simulink model "Convolution_Stream_Ex2"  (R2025a)
settings: Solver=ode4  StopTime=10
undefined symbols (not defined in the file): S, Valid, vsva2197, xcvc1902
libraries: aieUtilities x2, aieDSP x1, vmcUtilities x1
settings Model: Creator=sais  LastModifiedBy=robg

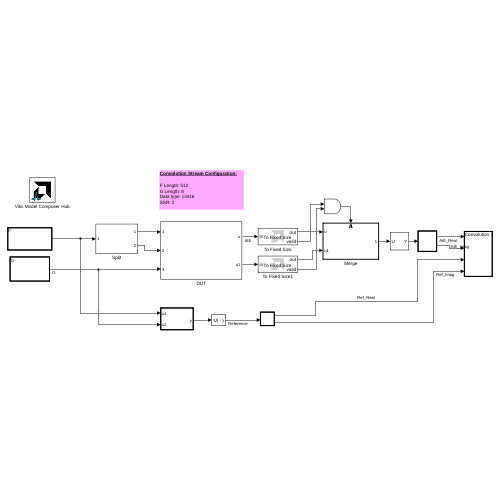
[thumbnail: Simulink's stored preview of the top-level diagram]
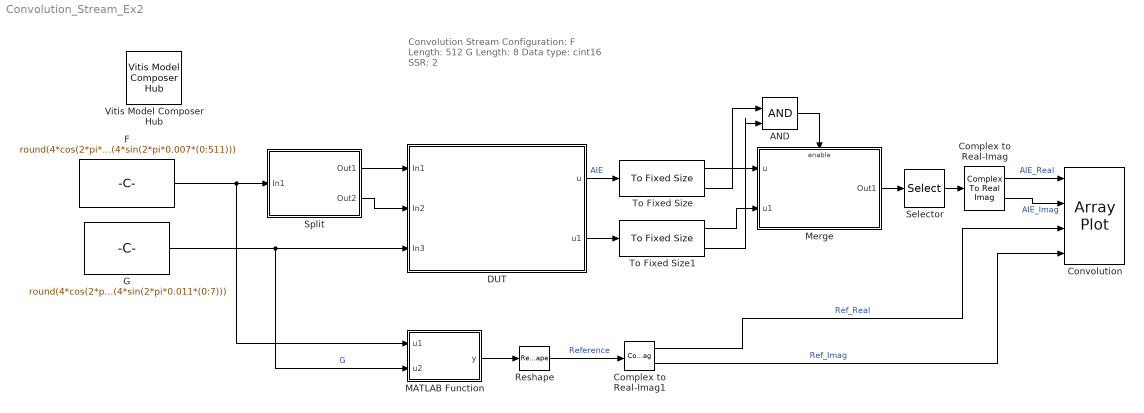
== system Convolution_Stream_Ex2 ==
  note: Convolution Stream Configuration:
      |
      | F Length: 512
      | G Length: 8
      | Data type: cint16
      | SSR: 2
  AND : Logic  IconShape=distinctive  AllPortsSameDT=off  OutDataTypeStr=boolean
  Complex to Real-Imag : ComplexToRealImag
  Complex to Real-Imag1 : ComplexToRealImag
  Convolution : ArrayPlot  NumInputPorts=4  WindowPosition=[379.000000,271.000000,1269.000000,725.000000,]  Visible=on  ScopeFrameLocation=window  YLimits=[-185 185]  ShowLegend=on
  DUT : Subsystem
  F : Constant  Value=round(4*cos(2*pi*0.013*(0:511))) + 1i*round(4*sin(2*pi*0.007*(0:511)))  OutDataTypeStr=int16  SampleTime=1
  G : Constant  Value=round(4*cos(2*pi*0.02*(0:7))) + 1i*round(4*sin(2*pi*0.011*(0:7)))  VectorParams1D=off  OutDataTypeStr=int16  SampleTime=1
  MATLAB Function : MATLAB Function  TreatAsAtomicUnit=on
  Merge : Subsystem
  Reshape : Reshape
  Selector : Selector  InputPortWidth=512  IndexOptions=Index vector (dialog)  Indices=1:1:512-8+1  OutputSizes=1
  Split : Subsystem
  To Fixed Size : aieUtilities/To Fixed Size  Mode=Produce a valid output signal  OutputSize=Inherit: Same as input  CopyMethod=Buffer samples to form output  HasStatusOutput=on
  To Fixed Size1 : aieUtilities/To Fixed Size  Mode=Produce a valid output signal  OutputSize=Inherit: Same as input  CopyMethod=Buffer samples to form output  HasStatusOutput=on
  Vitis Model Composer Hub : vmcUtilities/Vitis Model Composer Hub  Tag=genX  CodeGeneration=off  SubsystemName=DUT  BlockHierPath=Convolution_Stream_Ex2/DUT  CompilationType=HDLCompilation  SubsystemType=DUTNode  ExportTypeV2=IP Catalog  AIEArrayConfig=Use entire AIE array  StartColumn=1  NumberOfColumns=1  TargetDirectory=./code_2iterations  exportDesign=off  analyzeDesign=on  validateDesignOnHw=off  ExportType=AI Engines  IpVendor=xilinx.com  IpLibrary=hls  IpVersion=1.0  IpHWLanguage=Verilog  AieCompilerOptions={}  AieSimulatorOptions={}  CreateTestbench=on  TestbenchStackSize=10  RunRtlSim=off  RunCSim=off  RunAieSim=off  enableSimulationTimeout=on  enableGraphIterations=on  AieSimTimeout=50000  AieGraphIterations=-1  RunAieSimProfiling=off  LaunchVitisAnalyzer=off  PlotOutput=off  RunX86Sim=off  X86SimTimeout=10  GenHwImage=off  GenLibadfXo=off  GenHwValidationCode=off  PlatformType=Not Specified  HwSystemType=Baremetal  HwValidationTarget=hw  ProjDevice=xcvc1902-vsva2197-1LP-e-S  ProjDevicePart=xcvc1902-vsva2197-1LP-e-S  AIEType=AIE  SamplePeriod=-1  ClockFrequency=200  DataPathParallelism=1  xilinxfamily=versalaicore  part=xcvc1902  speed=-1LP-e-S  package=vsva2197  directory=./netlist  testbench=off  incr_netlist=off  synthesis_tool=Vivado  clock_wrapper=Clock Enables  dbl_ovrd=According to Block Masks  dcm_input_clock_period=10  sysclk_period=10  simulink_period=1  eval_field=0  IPInfoJsonString="{\"DUTSubsystemName\":\"DUT\",\"AIESubsystem\":{\"SubsystemName\":\"DUT\",\"TargetDirectory\":\"./code_2iterations\",\"AIEArrayConfig\":\"Use entire AIE array\",\"StartColumn\":\"0\",\"NumberOfColumns\":\"1\"},\"SubsystemTag\":\"AIENode\"}"  LogFileName=''  NThreads=4  IPConfigFile=/tmp/vmctmp-11698742404697829623/stream_correlation_smoke_ipconfig.json
  wires:
  MATLAB Function/1(y) -> Reshape/1
  Reshape/1 -> Complex to Real-Imag1/1  "Reference"
  Complex to Real-Imag/1 -> Convolution/1  "AIE_Real"
  Complex to Real-Imag/2 -> Convolution/2  "AIE_Imag"
  Complex to Real-Imag1/2 -> Convolution/4  "Ref_Imag"
  Complex to Real-Imag1/1 -> Convolution/3  "Ref_Real"
  F/1 -> MATLAB Function/1(u1), Split/1(In1)
  Split/1(Out1) -> DUT/1(In1)
  Split/2(Out2) -> DUT/2(In2)
  Merge/1(Out1) -> Selector/1
  DUT/1(u) -> To Fixed Size/1  "AIE"
  G/1 -> MATLAB Function/2(u2), DUT/3(In3)  "G"
  To Fixed Size/1 -> Merge/1(u)
  AND/1 -> Merge/Enable
  To Fixed Size/2 -> AND/1
  DUT/2(u1) -> To Fixed Size1/1
  To Fixed Size1/1 -> Merge/2(u1)
  To Fixed Size1/2 -> AND/2
  Selector/1 -> Complex to Real-Imag/1

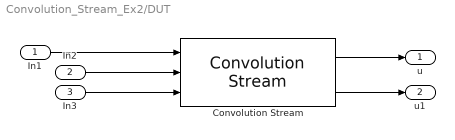
== system Convolution_Stream_Ex2/DUT ==
  In1 : Inport
  In2 : Inport  Port=2
  In3 : Inport  Port=3
  Convolution Stream : aieDSP/Convolution Stream  AIE_VARIANT=1  api=1  data_type_f=cint16  data_type_g=cint16  data_type_out=cint16  function_type=1  compute_mode=Valid (2)  f_sample_size=512  g_sample_size=8  USE_RTP_VECTOR_LENGTHS=off  num_frames=1  shift_output=0  rnd_mode=Floor  sat_mode=None  no_of_kernels=2  casc_length=1  blockJsonConstraints=[]  blockJsonConstraintsInternal=[]  spec=vmc_stream_conv.json  SerializedMaskParamNames=[]  SerializedMaskParamValues=[]  SerializedMaskParamVisibilities=[]  block_type=Convolution Stream  SerializedMaskParamDataypes=uint|uint|typename|typename|typename|uint|uint|uint|uint|uint|uint|uint|uint|uint|uint|uint  SerializedMaskParamEnumStrArr=0|0|0|0|0|0|Valid (2)|0|0|0|0|0|Floor,Ceiling,Round to positive infinity,Round to negative infinity,Round symmetrical to infinity,Round symmetrical to zero,Round convergent to even,Round convergent to odd|None,Saturate,Symmetric|0|0  SerializedMaskParamEnumValArr=0|0|0|0|0|0|2|0|0|0|0|0|0,1,2,3,4,5,6,7|0,1,3|0|0  SerializedMaskParamVectorArr=0|0|0|0|0|0|0|0|0|0|0|0|0|0|0|0  SerializedMaskParamKeys=AIE_VARIANT|TP_API|TT_DATA_F|TT_DATA_G|TT_DATA_OUT|TP_FUNCT_TYPE|TP_COMPUTE_MODE|TP_F_LEN|TP_G_LEN|TP_USE_RTP_VECTOR_LENGTHS|TP_NUM_FRAMES|TP_SHIFT|TP_RND|TP_SAT|TP_PHASES|TP_CASC_LEN
  u : Outport
  u1 : Outport  Port=2
  wires:
  In1/1 -> Convolution Stream/1
  Convolution Stream/1 -> u/1
  In2/1 -> Convolution Stream/2
  In3/1 -> Convolution Stream/3
  Convolution Stream/2 -> u1/1

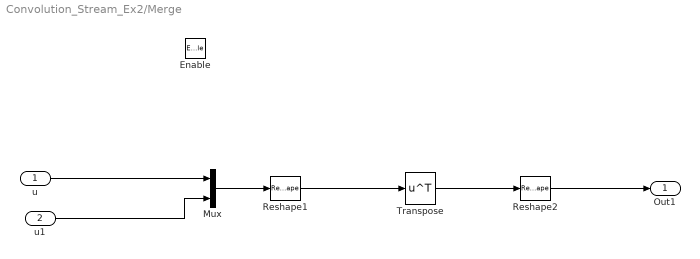
== system Convolution_Stream_Ex2/Merge ==
  u : Inport
  u1 : Inport  Port=2
  Enable : EnablePort
  Mux : Mux  Inputs=2
  Reshape1 : Reshape  OutputDimensionality=Customize  OutputDimensions=[256, 2]
  Reshape2 : Reshape  OutputDimensions=[1, 10]
  Transpose : Math  Operator=transpose
  Out1 : Outport
  wires:
  Reshape1/1 -> Transpose/1
  u/1 -> Mux/1
  Mux/1 -> Reshape1/1
  Transpose/1 -> Reshape2/1
  u1/1 -> Mux/2
  Reshape2/1 -> Out1/1

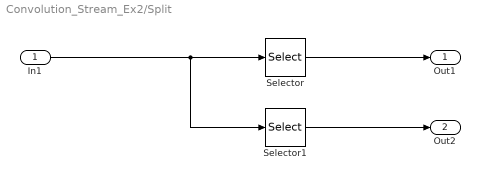
== system Convolution_Stream_Ex2/Split ==
  In1 : Inport
  Selector : Selector  InputPortWidth=512  IndexOptions=Index vector (dialog)  Indices=1:2:512  OutputSizes=1
  Selector1 : Selector  InputPortWidth=512  IndexOptions=Index vector (dialog)  Indices=2:2:512  OutputSizes=1
  Out1 : Outport
  Out2 : Outport  Port=2
  wires:
  In1/1 -> Selector/1, Selector1/1
  Selector1/1 -> Out2/1
  Selector/1 -> Out1/1

== matlab function Convolution_Stream_Ex2/MATLAB Function ==
  data: u1 input; y output; u2 input
function y = fcn(u1,u2)

y = int16(conv(u1,u2,"valid"));
